simulink model "P2_Muestreo_Uniforme"  (R2020a)
settings: Solver=FixedStepDiscrete  StartTime=0.0  StopTime=25  FixedStep=0.001  RelTol=1e-3
settings Model: Creator=León Mora  LastModifiedBy=León Mora

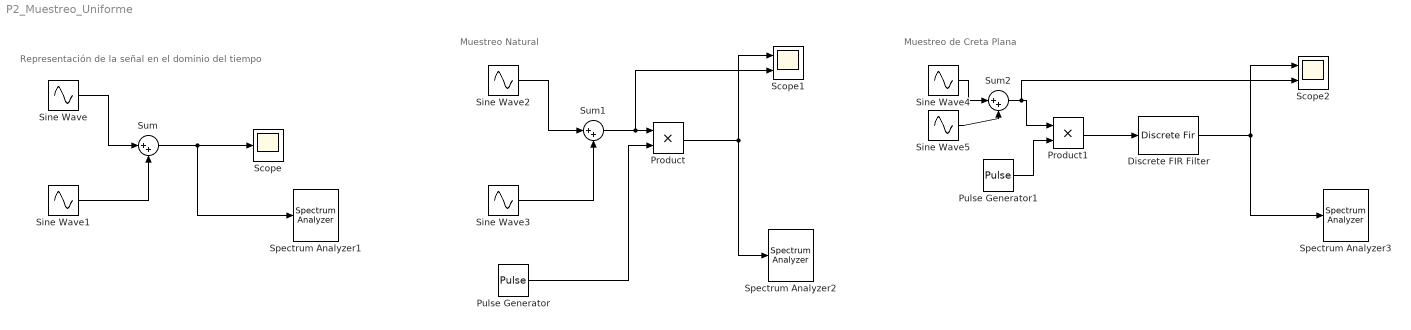
== system P2_Muestreo_Uniforme ==
  note: Muestreo de Creta Plana
  note: Muestreo Natural
  note: Representación de la señal en el dominio del tiempo
  Discrete FIR Filter : DiscreteFir  Coefficients=ones(1,25)  SampleTime=1e-3
  Product : Product
  Product1 : Product
  Pulse Generator : DiscretePulseGenerator  PulseType=Time based  Period=0.1  PulseWidth=25
  Pulse Generator1 : DiscretePulseGenerator  PulseType=Time based  Period=0.1
  Scope : Scope
  Scope1 : Scope  NumInputPorts=2
  Scope2 : Scope  NumInputPorts=2
  Sine Wave : Sin  Frequency=2*pi  SampleTime=1e-3
  Sine Wave1 : Sin  Frequency=6*pi  SampleTime=1e-3
  Sine Wave2 : Sin  Frequency=2*pi  SampleTime=1e-3
  Sine Wave3 : Sin  Frequency=6*pi  SampleTime=1e-3
  Sine Wave4 : Sin  Frequency=2*pi  SampleTime=1e-3
  Sine Wave5 : Sin  Frequency=6*pi  SampleTime=1e-3
  Spectrum Analyzer1 : SpectrumAnalyzer
  Spectrum Analyzer2 : SpectrumAnalyzer
  Spectrum Analyzer3 : SpectrumAnalyzer
  Sum : Sum  Inputs=|++
  Sum1 : Sum  Inputs=|++
  Sum2 : Sum  Inputs=|++
  wires:
  Sine Wave1/1 -> Sum/2
  Sine Wave/1 -> Sum/1
  Sum/1 -> Scope/1, Spectrum Analyzer1/1
  Sine Wave3/1 -> Sum1/2
  Sine Wave2/1 -> Sum1/1
  Pulse Generator/1 -> Product/2
  Sum1/1 -> Scope1/2, Product/1
  Product/1 -> Spectrum Analyzer2/1, Scope1/1
  Sine Wave4/1 -> Sum2/1
  Sine Wave5/1 -> Sum2/2
  Sum2/1 -> Scope2/2, Product1/1
  Pulse Generator1/1 -> Product1/2
  Discrete FIR Filter/1 -> Spectrum Analyzer3/1, Scope2/1
  Product1/1 -> Discrete FIR Filter/1
